simulink model "regs_hdl_test"  (R2019b)
settings: Solver=FixedStepDiscrete  StartTime=0.0  StopTime=16  RelTol=1e-3
libraries: simulink x5, dspsigops x4, lib_dsphdlcontrol_v1 x3, dspsrcs4 x2
settings Model: DataTypeOverride=Off  Creator=mbabst  LastModifiedBy=mbabst
settings DataIOCC: SaveOutput=off  SaveTime=off
settings OptimizationCC: BlockReduction=off  ConditionallyExecuteInputs=off  DefaultParameterBehavior=Inlined  LifeSpan=inf
settings DebuggingCC: AlgebraicLoopMsg=error  SingleTaskRateTransMsg=error  StrictBusMsg=ErrorOnBusTreatedAsVector  SFUnexpectedBacktrackingDiag=warning  SFNoUnconditionalDefaultTransitionDiag=warning  SFExecutionAtInitializationDiag=none  ArithmeticOperatorsInVariantConditions=warning
settings HardwareCC: ProdBitPerPointer=32  ProdBitPerSizeT=32  ProdBitPerPtrDiffT=32  ProdLargestAtomicFloat=None  ProdIntDivRoundTo=Undefined  ProdEndianess=Unspecified  ProdWordSize=32  ProdHWDeviceType=ASIC/FPGA->ASIC/FPGA  ProdEqTarget=off
settings SFSimCC: SimUseLocalCustomCode=off  CustomCodeUndefinedFunction=UseInterfaceOnly
settings RTWCC: RTWUseLocalCustomCode=off
settings CodeAppCC: StateflowObjectComments=on
settings GRTTargetCC: TargetLangStandard=C89/C90 (ANSI)
settings ConfigComp: CovMetricSettings=dw  CovHtmlReporting=on  CovSaveCumulativeToWorkspaceVar=on  CovSaveSingleToWorkspaceVar=on  CovExternalEMLEnable=off

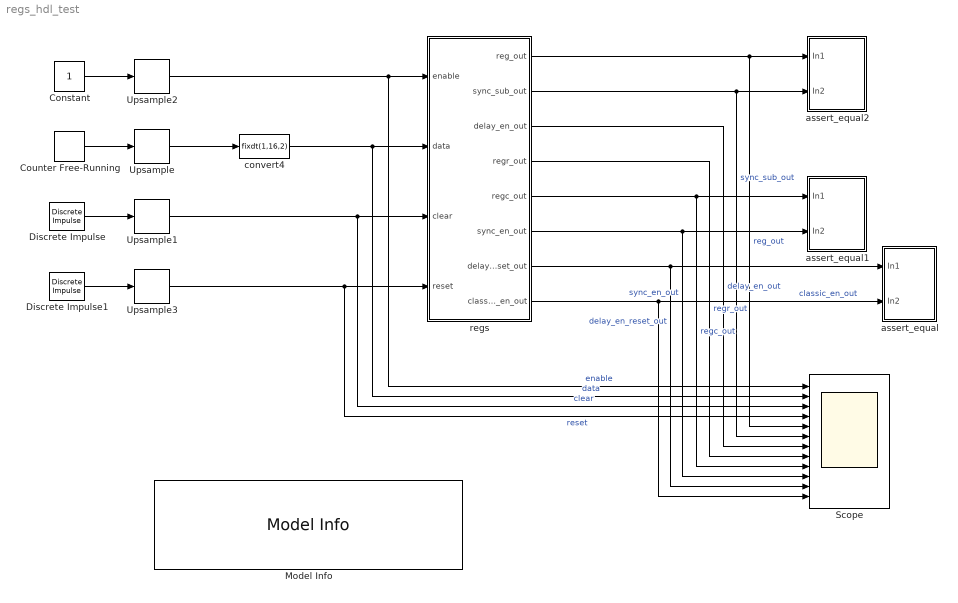
== system regs_hdl_test ==
  Constant : Constant  OutDataTypeStr=boolean  SampleTime=-1
  Counter Free-Running : simulink/Sources/Counter Free-Running  NumBits=16  tsamp=-1
  Discrete Impulse : dspsrcs4/Discrete  Impulse  Delay=10  SampleTime=1  FrameSample=1  OutputFrames=off  dataType=boolean  isSigned=on  wordLen=16  udDataType=sfix(16)  fracBitsMode=Best precision  numFracBits=15  OutDataTypeStr=boolean  LastOutDataTypeStr=boolean
  Discrete Impulse1 : dspsrcs4/Discrete  Impulse  Delay=10  SampleTime=1  FrameSample=1  OutputFrames=off  dataType=boolean  isSigned=on  wordLen=16  udDataType=sfix(16)  fracBitsMode=Best precision  numFracBits=15  OutDataTypeStr=boolean  LastOutDataTypeStr=boolean
  Model Info : simulink/Model-Wide Utilities/Model Info  Frame=on  DisplayStringWithTags=|  HorizontalTextAlignment=Left  LeftAlignmentValue=0.02
      | Copyright (c) 2005-2021 DSPlogic, Inc.
      | Distributed under the terms of the Simplified BSD License.
      | The full license is in the file LICENSE, distributed with this software.
      | 
      | Model: %<ModelName> (v%<ModelVersion>)
      | Author: Michael Babst <mike.babst@dsplogic.com>
      | Created: by %<Creator> on %<Created>
      | Modified: by %<ModifiedBy> on %<LastModificationDate>
  Scope : Scope  NumInputPorts=12
  Upsample{,1..3} (4 alike) : dspsigops/Upsample  N=4  phase=0  RateOptions=Allow multirate processing  ic=0  mode=Unused parameter value
  assert_equal : Subsystem
  assert_equal1 : Subsystem
  assert_equal2 : Subsystem
  convert4 : DataTypeConversion  OutDataTypeStr=fixdt(1,16,2)  SaturateOnIntegerOverflow=on
  regs : Subsystem
  wires:
  Discrete Impulse/1 -> Upsample1/1
  Constant/1 -> Upsample2/1
  Counter Free-Running/1 -> Upsample/1
  Upsample/1 -> convert4/1
  convert4/1 -> Scope/2, regs/2(data)  "data"
  Upsample2/1 -> Scope/1, regs/1(enable)  "enable"
  Upsample1/1 -> regs/3(clear), Scope/3  "clear"
  Discrete Impulse1/1 -> Upsample3/1
  Upsample3/1 -> regs/4(reset), Scope/4  "reset"
  regs/1(reg_out) -> assert_equal2/1(In1), Scope/5  "reg_out"
  regs/4(regr_out) -> Scope/8  "regr_out"
  regs/3(delay_en_out) -> Scope/7  "delay_en_out"
  regs/7(delay_en_reset_out) -> assert_equal/1(In1), Scope/11  "delay_en_reset_out"
  regs/6(sync_en_out) -> assert_equal1/2(In2), Scope/10  "sync_en_out"
  regs/8(classic_en_out) -> assert_equal/2(In2), Scope/12  "classic_en_out"
  regs/5(regc_out) -> assert_equal1/1(In1), Scope/9  "regc_out"
  regs/2(sync_sub_out) -> assert_equal2/2(In2), Scope/6  "sync_sub_out"

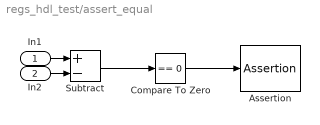
== system regs_hdl_test/assert_equal ==
  In1 : Inport
  In2 : Inport  Port=2
  Assertion : Assertion
  Compare To Zero : simulink/Logic and Bit Operations/Compare To Zero  relop===  OutDataTypeStr=boolean
  Subtract : Sum  Inputs=+-
  wires:
  In2/1 -> Subtract/2
  Subtract/1 -> Compare To Zero/1
  Compare To Zero/1 -> Assertion/1
  In1/1 -> Subtract/1

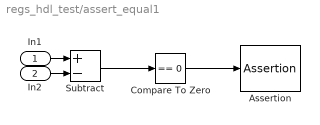
== system regs_hdl_test/assert_equal1 ==
  In1 : Inport
  In2 : Inport  Port=2
  Assertion : Assertion
  Compare To Zero : simulink/Logic and Bit Operations/Compare To Zero  relop===  OutDataTypeStr=boolean
  Subtract : Sum  Inputs=+-
  wires:
  In2/1 -> Subtract/2
  Subtract/1 -> Compare To Zero/1
  Compare To Zero/1 -> Assertion/1
  In1/1 -> Subtract/1

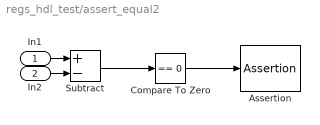
== system regs_hdl_test/assert_equal2 ==
  In1 : Inport
  In2 : Inport  Port=2
  Assertion : Assertion
  Compare To Zero : simulink/Logic and Bit Operations/Compare To Zero  relop===  OutDataTypeStr=boolean
  Subtract : Sum  Inputs=+-
  wires:
  In2/1 -> Subtract/2
  Subtract/1 -> Compare To Zero/1
  Compare To Zero/1 -> Assertion/1
  In1/1 -> Subtract/1

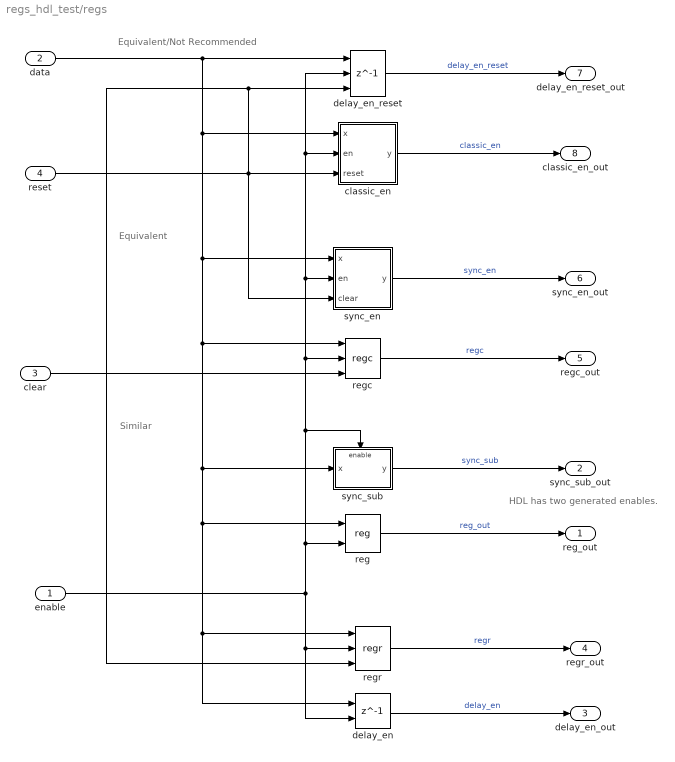
== system regs_hdl_test/regs ==
  note: HDL has two generated enables.
  note: Equivalent/Not Recommended
  note: Equivalent
  note: Similar
  enable : Inport
  data : Inport  Port=2
  clear : Inport  Port=3
  reset : Inport  Port=4
  classic_en : Subsystem
  delay_en : Delay  DelayLength=1  ShowEnablePort=on
      settings: InputPortMap=u0,e6
  delay_en_reset : Delay  DelayLength=1  ExternalReset=Level  ShowEnablePort=on
      settings: InputPortMap=u0,e6,r5
  reg : lib_dsphdlcontrol_v1/reg  vinit=0.0  tsamp=-1
      settings: SourceProductName=DSPHDL Library
  regc : lib_dsphdlcontrol_v1/regc  vinit=0.0  tsamp=-1
      settings: SourceProductName=DSPHDL Library
  regr : lib_dsphdlcontrol_v1/regr  vinit=0.0  tsamp=-1
      settings: SourceProductName=DSPHDL Library
  sync_en : Subsystem
  sync_sub : Subsystem
  reg_out : Outport
  sync_sub_out : Outport  Port=2
  delay_en_out : Outport  Port=3
  regr_out : Outport  Port=4
  regc_out : Outport  Port=5
  sync_en_out : Outport  Port=6
  delay_en_reset_out : Outport  Port=7
  classic_en_out : Outport  Port=8
  wires:
  data/1 -> delay_en/1, regr/1, reg/1, sync_sub/1(x), regc/1, sync_en/1(x), classic_en/1(x), delay_en_reset/1
  reset/1 -> regr/3, delay_en_reset/3, sync_en/3(clear), classic_en/3(reset)
  enable/1 -> sync_sub/Enable, sync_en/2(en), classic_en/2(en), delay_en_reset/2, regc/2, reg/2, delay_en/2, regr/2
  reg/1 -> reg_out/1  "reg_out"
  regr/1 -> regr_out/1  "regr"
  delay_en/1 -> delay_en_out/1  "delay_en"
  delay_en_reset/1 -> delay_en_reset_out/1  "delay_en_reset"
  sync_en/1(y) -> sync_en_out/1  "sync_en"
  clear/1 -> regc/3
  classic_en/1(y) -> classic_en_out/1  "classic_en"
  regc/1 -> regc_out/1  "regc"
  sync_sub/1(y) -> sync_sub_out/1  "sync_sub"

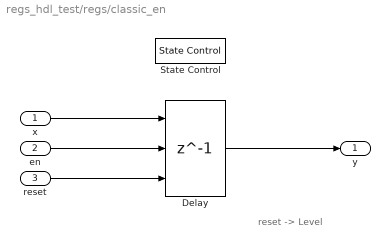
== system regs_hdl_test/regs/classic_en ==
  note: reset -> Level
  x : Inport
  en : Inport  Port=2
  reset : Inport  Port=3
  Delay : Delay  DelayLength=1  ExternalReset=Level  ShowEnablePort=on
      settings: InputPortMap=u0,e6,r5
  State Control : StateControl
  y : Outport
  wires:
  x/1 -> Delay/1
  reset/1 -> Delay/3
  Delay/1 -> y/1
  en/1 -> Delay/2

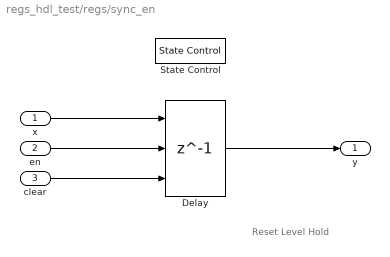
== system regs_hdl_test/regs/sync_en ==
  note: Reset Level Hold
  x : Inport
  en : Inport  Port=2
  clear : Inport  Port=3
  Delay : Delay  DelayLength=1  ExternalReset=Level hold  ShowEnablePort=on
      settings: InputPortMap=u0,e6,r5
  State Control : StateControl  StateControl=Synchronous
  y : Outport
  wires:
  x/1 -> Delay/1
  clear/1 -> Delay/3
  Delay/1 -> y/1
  en/1 -> Delay/2

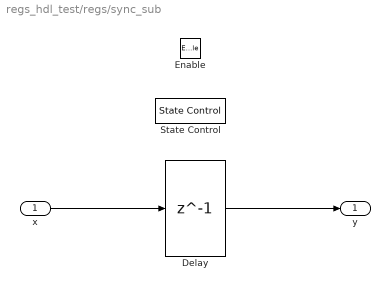
== system regs_hdl_test/regs/sync_sub ==
  x : Inport
  Enable : EnablePort
  Delay : Delay  DelayLength=1
  State Control : StateControl  StateControl=Synchronous
  y : Outport
  wires:
  x/1 -> Delay/1
  Delay/1 -> y/1
